simulink model "sim_x"  (R2019b)
settings: Solver=VariableStepAuto  StartTime=0.0  StopTime=10.0  RelTol=1e-3
settings Model: Creator=vidma  LastModifiedBy=vidma

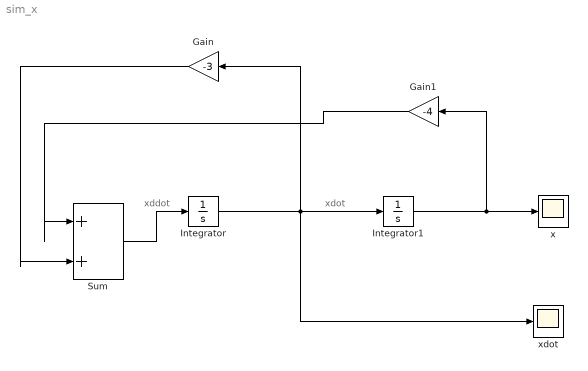
== system sim_x ==
  note: xdot
  note: xddot
  Gain : Gain  Gain=-3
  Gain1 : Gain  Gain=-4
  Integrator : Integrator
  Integrator1 : Integrator  InitialCondition=1
  Sum : Sum  Inputs=|++
  x : Scope
  xdot : Scope
  wires:
  Integrator1/1 -> Gain1/1, x/1
  Gain1/1 -> Sum/1
  Integrator/1 -> xdot/1, Gain/1, Integrator1/1
  Gain/1 -> Sum/2
  Sum/1 -> Integrator/1
